simulink model "IEEE10_decommision"  (R2015b)
settings: Solver=FixedStepAuto  StartTime=0.0  StopTime=30  FixedStep=Ts  RelTol=1e-3
undefined symbols (not defined in the file): Cbase, Lbase, Ts, Xbase
libraries: powerlib x150, powerlib_meascontrol x27, simulink x9, sps_avr x3, powerlib_extras x1
(part 1 of 2)
settings Model: SimulationMode=accelerator  Creator=Eren  LastModifiedBy=Eren
settings DebuggingCC: UnconnectedInputMsg=none  UnconnectedOutputMsg=none  UnconnectedLineMsg=none

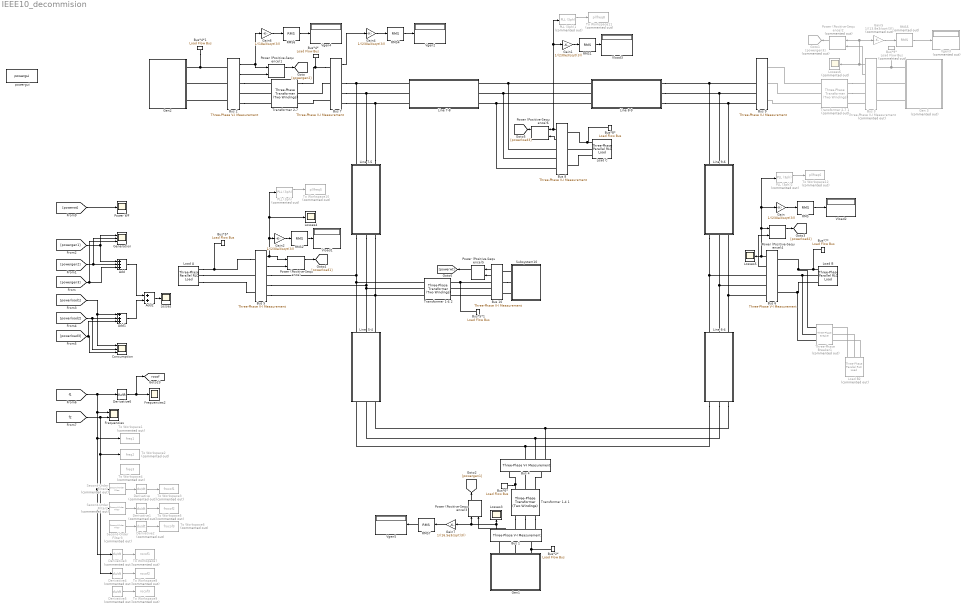
== system IEEE10_decommision ==
  Add : Sum  Inputs=3
  Add1 : Sum  Inputs=3
  Add2 : Sum
  Bus {1..2,4..10} (9 alike) : powerlib/Measurements/Three-Phase V-I Measurement  VoltageMeasurement=phase-to-ground  SetLabelV=off  LabelV=Vsabc  Vpu=off  VpuLL=on  CurrentMeasurement=yes  SetLabelI=off  LabelI=Isabc  Ipu=off  Pbase=100e6  Vbase=690  OutputType=Complex  PhasorSimulation=off  PSBequivalent=0
  Bus 3 : powerlib/Measurements/Three-Phase V-I Measurement  Commented=on  VoltageMeasurement=phase-to-ground  SetLabelV=off  LabelV=Vsabc  Vpu=off  VpuLL=on  CurrentMeasurement=yes  SetLabelI=off  LabelI=Isabc  Ipu=off  Pbase=100e6  Vbase=690  OutputType=Complex  PhasorSimulation=off  PSBequivalent=0
  Bus*2* : powerlib/Measurements/Load Flow Bus  LConnTagsString=a  Phases=single  Connectors=on one side  ID=Bus*1*  Vbase=16500  Vref=1.04  Vangle=0  VLF=1.04  VLFb=1  VLFc=1  angleLF=0  angleLFb=0  angleLFc=0
  Bus*4* : powerlib/Measurements/Load Flow Bus  LConnTagsString=a  Phases=single  Connectors=on one side  ID=Bus*7*  Vbase=230000  Vref=1  Vangle=0  VLF=1.027  VLFb=1  VLFc=1  angleLF=-1.988  angleLFb=0  angleLFc=0
  Bus*4*1 : powerlib/Measurements/Load Flow Bus  LConnTagsString=a  Phases=single  Connectors=on one side  ID=Bus*2*  Vbase=18e3  Vref=1.025  Vangle=0  VLF=1.025  VLFb=1  VLFc=1  angleLF=3.56  angleLFb=0  angleLFc=0
  Bus*5* : powerlib/Measurements/Load Flow Bus  LConnTagsString=a  Phases=single  Connectors=on one side  ID=Bus*5*  Vbase=230e3  Vref=1  Vangle=0  VLF=1.013  VLFb=1  VLFc=1  angleLF=-6.161  angleLFb=0  angleLFc=0
  Bus*5*1 : powerlib/Measurements/Load Flow Bus  LConnTagsString=a  Phases=single  Connectors=on one side  ID=Bus*10*  Vbase=690  Vref=1  Vangle=0  VLF=1.013  VLFb=1  VLFc=1  angleLF=-6.164  angleLFb=0  angleLFc=0
  Bus*6* : powerlib/Measurements/Load Flow Bus  LConnTagsString=a  Phases=single  Connectors=on one side  ID=Bus*4*  Vbase=230000  Vref=1  Vangle=0  VLF=1.034  VLFb=1  VLFc=1  angleLF=-4.035  angleLFb=0  angleLFc=0
  Bus*7* : powerlib/Measurements/Load Flow Bus  LConnTagsString=a  Phases=single  Connectors=on one side  ID=Bus*6*  Vbase=230e3  Vref=1  Vangle=0  VLF=1.022  VLFb=1  VLFc=1  angleLF=-8.159  angleLFb=0  angleLFc=0
  Bus*8* : powerlib/Measurements/Load Flow Bus  LConnTagsString=a  Phases=single  Connectors=on one side  ID=Bus*8*  Vbase=230e3  Vref=1  Vangle=0  VLF=1.018  VLFb=1  VLFc=1  angleLF=-6.531  angleLFb=0  angleLFc=0
  Bus*9* : powerlib/Measurements/Load Flow Bus  Commented=on  LConnTagsString=a  Phases=single  Connectors=on one side  ID=Bus*3*  Vbase=13800  Vref=1.025  Vangle=0  VLF=1.025  VLFb=1  VLFc=1  angleLF=6.455  angleLFb=0  angleLFc=0
  Concumption : Scope  NumInputPorts=3
  Derivative{,1..5} (6 alike) : Derivative  Commented=on
  Derivative6 : Derivative
  Frequencies : Scope  NumInputPorts=2
  Frequencies2 : Scope
  Gain{,1..2,4} (4 alike) : Gain  Gain=1/(230e3/sqrt(3))
  Gain5 : Gain  Commented=on  Gain=1/(13.8e3/sqrt(3))
  Gain6 : Gain  Gain=1/(18e3/sqrt(3))
  Gain7 : Gain  Gain=1/(16.5e3/sqrt(3))
  Gen 3 : Subsystem  Commented=on
  Gen1 : Subsystem
  Gen2 : Subsystem
  "Generation " : Scope  NumInputPorts=3
  Goto1 : Goto  Commented=on  GotoTag=powergen3
  Line  5-4 : Subsystem
  Line 6-4 : Subsystem
  Line 7-5 : Subsystem
  Line 7-8 : Subsystem
  Line 8-9 : Subsystem
  Line 9-6 : Subsystem
  Load A : powerlib/Elements/Three-Phase Parallel RLC Load  LConnTagsString=A|B|C  Configuration=Y (grounded)  NominalVoltage=(230000)*1.01282  Vabc=[1e3 1e3 1e3]  Vabcp=[1e3 1e3 1e3]  NominalFrequency=50  UnbalancedPower=off  ActivePower=125e6  InductivePower=50e6  CapacitivePower=0  Pabc=[10e3 9e3 11e3]  QLabc=[100 90 110]  QCabc=[100 90 110]  Pabcp=[10e3 9e3 11e3]  QLabcp=[100 90 110]  QCabcp=[100 90 110]  Measurements=None  LoadType=constant PQ
  Load B : powerlib/Elements/Three-Phase Parallel RLC Load  LConnTagsString=A|B|C  Configuration=Y (grounded)  NominalVoltage=(230000)*1.0221  Vabc=[1e3 1e3 1e3]  Vabcp=[1e3 1e3 1e3]  NominalFrequency=50  UnbalancedPower=off  ActivePower=90e6  InductivePower=30e6  CapacitivePower=0  Pabc=[10e3 9e3 11e3]  QLabc=[100 90 110]  QCabc=[100 90 110]  Pabcp=[10e3 9e3 11e3]  QLabcp=[100 90 110]  QCabcp=[100 90 110]  Measurements=None  LoadType=constant PQ
  Load B2 : powerlib/Elements/Three-Phase Parallel RLC Load  Commented=on  LConnTagsString=A|B|C  Configuration=Y (grounded)  NominalVoltage=230e3  Vabc=[1e3 1e3 1e3]  Vabcp=[1e3 1e3 1e3]  NominalFrequency=50  UnbalancedPower=off  ActivePower=31.5e6*2  InductivePower=0  CapacitivePower=0  Pabc=[10e3 9e3 11e3]  QLabc=[100 90 110]  QCabc=[100 90 110]  Pabcp=[10e3 9e3 11e3]  QLabcp=[100 90 110]  QCabcp=[100 90 110]  Measurements=None  LoadType=constant PQ
  Load C : powerlib/Elements/Three-Phase Parallel RLC Load  LConnTagsString=A|B|C  Configuration=Y (grounded)  NominalVoltage=(230000)*1.01809  Vabc=[1e3 1e3 1e3]  Vabcp=[1e3 1e3 1e3]  NominalFrequency=50  UnbalancedPower=off  ActivePower=100e6  InductivePower=35e6  CapacitivePower=0  Pabc=[10e3 9e3 11e3]  QLabc=[100 90 110]  QCabc=[100 90 110]  Pabcp=[10e3 9e3 11e3]  QLabcp=[100 90 110]  QCabcp=[100 90 110]  Measurements=None  LoadType=constant PQ
  "Losses " : Scope
  Losses3 : Scope
  Losses4 : Scope
  Losses5 : Scope
  Losses6 : Scope  Commented=on
  PLL (3ph) : powerlib_meascontrol/PLL/PLL (3ph)  Commented=on  Fmin=45  Par_Init=[0, 50]  ParK=[180, 3200, 1]  TcD=1e-4  MaxRateChangeFreq=12  FilterCutOffFreq=25  Ts=0  AGC=on
  PLL (3ph)1 : powerlib_meascontrol/PLL/PLL (3ph)  Commented=on  Fmin=45  Par_Init=[0, 50]  ParK=[180, 3200, 1]  TcD=1e-4  MaxRateChangeFreq=12  FilterCutOffFreq=25  Ts=0  AGC=on
  PLL (3ph)2 : powerlib_meascontrol/PLL/PLL (3ph)  Commented=on  Fmin=45  Par_Init=[0, 50]  ParK=[180, 3200, 1]  TcD=1e-4  MaxRateChangeFreq=12  FilterCutOffFreq=25  Ts=0  AGC=on
  Power (Positive-Sequence){,1,3..6} (6 alike) : powerlib_meascontrol/Measurements/Power (Positive-Sequence)  Freq=50  Vinit=[0, 0]  Iinit=[0, 0]  Ts=0
  Power (Positive-Sequence)2 : powerlib_meascontrol/Measurements/Power (Positive-Sequence)  Commented=on  Freq=50  Vinit=[0, 0]  Iinit=[0, 0]  Ts=0
  Power WF : Scope
  RMS{,1..2,4,6..7} (6 alike) : powerlib_meascontrol/Measurements/RMS  TrueRMS=on  Freq=50  RMSInit=120  Ts=0
  RMS5 : powerlib_meascontrol/Measurements/RMS  Commented=on  TrueRMS=on  Freq=50  RMSInit=120  Ts=0
  Second-Order Filter1 : powerlib_meascontrol/Filters/Second-Order Filter  Commented=on  FilterType=Lowpass  Fo=2  Zeta=0.707  Ts=0  Initialize=off  Vac_Init="[0,  0,  60]"  Vdc_Init=0  PlotResponse=off  FreqRange=[0, 500, 1]
  Second-Order Filter2 : powerlib_meascontrol/Filters/Second-Order Filter  Commented=on  FilterType=Lowpass  Fo=2  Zeta=0.707  Ts=0  Initialize=off  Vac_Init="[0,  0,  60]"  Vdc_Init=0  PlotResponse=off  FreqRange=[0, 500, 1]
  Second-Order Filter3 : powerlib_meascontrol/Filters/Second-Order Filter  Commented=on  FilterType=Lowpass  Fo=2  Zeta=0.707  Ts=0  Initialize=off  Vac_Init="[0,  0,  60]"  Vdc_Init=0  PlotResponse=off  FreqRange=[0, 500, 1]
  Subsystem10 : Subsystem
  Three-Phase Breaker1 : powerlib/Elements/Three-Phase Breaker  Commented=on  InitialState=open  SwitchA=on  SwitchB=on  SwitchC=on  SwitchTimes=loadconnection  External=off  BreakerResistance=0.01  SnubberResistance=1e6  SnubberCapacitance=inf  Measurements=None
  To Workspace1 : ToWorkspace  Commented=on  VariableName=freq1  SaveFormat=Timeseries  SampleTime=-1
  To Workspace10 : ToWorkspace  Commented=on  VariableName=pllfreq5  SaveFormat=Timeseries  SampleTime=-1
  To Workspace11 : ToWorkspace  Commented=on  VariableName=pllfreq8  SaveFormat=Timeseries  SampleTime=-1
  To Workspace12 : ToWorkspace  Commented=on  VariableName=pllfreq6  SaveFormat=Timeseries  SampleTime=-1
  To Workspace2 : ToWorkspace  Commented=on  VariableName=freq2  SaveFormat=Timeseries  SampleTime=-1
  To Workspace3 : ToWorkspace  Commented=on  VariableName=frocof1  SaveFormat=Timeseries  SampleTime=-1
  To Workspace4 : ToWorkspace  Commented=on  VariableName=freq3  SaveFormat=Timeseries  SampleTime=-1
  To Workspace5 : ToWorkspace  Commented=on  VariableName=frocof2  SaveFormat=Timeseries  SampleTime=-1
  To Workspace6 : ToWorkspace  Commented=on  VariableName=frocof3  SaveFormat=Timeseries  SampleTime=-1
  To Workspace7 : ToWorkspace  Commented=on  VariableName=rocof1  SaveFormat=Timeseries  SampleTime=-1
  To Workspace8 : ToWorkspace  Commented=on  VariableName=rocof2  SaveFormat=Timeseries  SampleTime=-1
  To Workspace9 : ToWorkspace  Commented=on  VariableName=rocof3  SaveFormat=Timeseries  SampleTime=-1
  Transformer 1-4 1 : powerlib/Elements/Three-Phase Transformer (Two Windings)  Winding1Connection=Yg  Winding2Connection=Yg  CoreType=Three single-phase transformers  SetSaturation=off  Hysteresis=off  DataFile='hysteresis'  SetInitialFlux=off  Measurements=None  UNITS=pu  NominalPower=[ 250e6 , 50 ]  Winding1=[ 16.5e3 , 0.00001 , 0.144/2 ]  Winding2="[ 230e3 , 0.00001  , 0.144/2 ]"  Rm=500  Lm=500  L0=0.5  Saturation=[ 0,0 ; 0.0024,1.2 ; 1.0,1.52 ]  InitialFluxes=[ 0.8 , -0.8 , 0.7 ]  MoreParameters=off  BreakLoop=off  DataType=off  TransfoNumber=1
  Transformer 1-4 2 : powerlib/Elements/Three-Phase Transformer (Two Windings)  Winding1Connection=Yg  Winding2Connection=Yg  CoreType=Three single-phase transformers  SetSaturation=off  Hysteresis=off  DataFile='hysteresis'  SetInitialFlux=off  Measurements=None  UNITS=pu  NominalPower=[ 50e6 , 50 ]  Winding1=[ 690 , 0.00001 , 0.05/2 ]  Winding2="[ 230e3 , 0.00001  , 0.05/2 ]"  Rm=500  Lm=500  L0=0.5  Saturation=[ 0,0 ; 0.0024,1.2 ; 1.0,1.52 ]  InitialFluxes=[ 0.8 , -0.8 , 0.7 ]  MoreParameters=off  BreakLoop=off  DataType=off  TransfoNumber=1
  "Transformer 2-7 " : powerlib/Elements/Three-Phase Transformer (Two Windings)  Winding1Connection=Yg  Winding2Connection=Yg  CoreType=Three single-phase transformers  SetSaturation=off  Hysteresis=off  DataFile='hysteresis'  SetInitialFlux=off  Measurements=None  UNITS=pu  NominalPower=[ 200e6 , 50 ]  Winding1=[18000 1e-05 0.0625]  Winding2=[2.3e+05 1e-05 0.0625]  Rm=500  Lm=500  L0=0.5  Saturation=[0 0;0.0024 1.2;1 1.52]  InitialFluxes=[0.79999 -0.79999 0.69999]  MoreParameters=off  BreakLoop=off  DataType=off  TransfoNumber=1
  Transformer 2-7 1 : powerlib/Elements/Three-Phase Transformer (Two Windings)  Commented=on  Winding1Connection=Yg  Winding2Connection=Yg  CoreType=Three single-phase transformers  SetSaturation=off  Hysteresis=off  DataFile='hysteresis'  SetInitialFlux=off  Measurements=None  UNITS=pu  NominalPower=[ 150e6 , 50 ]  Winding1="[ 13.8e3 , 0.00001 , 0.0879/2  ]"  Winding2="[ 230e3 , 0.00001  , 0.0879/2 ]"  Rm=500  Lm=500  L0=0.5  Saturation=[ 0,0 ; 0.0024,1.2 ; 1.0,1.52 ]  InitialFluxes=[ 0.8 , -0.8 , 0.7 ]  MoreParameters=off  BreakLoop=off  DataType=off  TransfoNumber=1
  Vgen2 : Display
      settings: Decimation=5
  Vgen3 : Display  Commented=on
      settings: Decimation=5
  Vgen4 : Display
      settings: Decimation=5
  Vgen5 : Display
      settings: Decimation=5
  Vload1 : Display
      settings: Decimation=5
  Vload2 : Display
      settings: Decimation=5
  Vload3 : Display
      settings: Decimation=5
  powergui : powerlib/powergui  Priority=2  SimulationMode=Discrete  SolverType=Tustin  SampleTime=Ts  frequency=50  SPID=on  DisableSnubberDevices=on  DisableRonSwitches=on  DisableVfSwitches=on  SwTol=0  DisplayEquations=off  Interpol=off  ExternalGateDelay=off  methode=off  Ts=0  FunctionMessages=off  echomessages=off  HookPort=off  EnableUseOfTLC=off  x0status=steady  frequencyindice=50  Pbase=100e6  ErrMax=0.0001  Iterations=50  UnitsV=kV  UnitsW=MW  buscounter=10  RestoreLinks=warning  ResistiveCurrentMeasurement=off  Frange=[0:2:500]  Ylog=off  Xlog=on  ShowGrid=off  save=off  variable=ZData  structure=0  ZoomFFT=on  StartTime=0.0  cycles=1  DisplayStyle=1  fundamental=60  FreqAxis=off  MaxFrequency=1000  frequencyindicesteady=1  RmsSteady=2  display=off
  tag scope: rocof=global
  wires:
  Bus 5/2 -> Power (Positive-Sequence)/2
  Power (Positive-Sequence)/1 -> [powerload1]
  Bus 2/2 -> Power (Positive-Sequence)1/2
  Bus 3/2 -> Power (Positive-Sequence)2/2
  Bus 1/2 -> Power (Positive-Sequence)3/2
  Power (Positive-Sequence)1/1 -> [powergen2]
  Power (Positive-Sequence)2/1 -> Goto1/1
  Power (Positive-Sequence)3/1 -> [powergen1]
  Bus 6/2 -> Power (Positive-Sequence)4/2
  Power (Positive-Sequence)4/1 -> [powerload2]
  [powergen1] -> "Generation "/1, Add/1
  [powergen2] -> Add/2, "Generation "/2
  [powergen3] -> "Generation "/3, Add/3
  [powerload1] -> Add1/1, Concumption/1
  [powerload2] -> Add1/2, Concumption/2
  [powerload3] -> Add1/3, Concumption/3
  Add/1 -> Add2/1
  Add1/1 -> Add2/2
  Add2/1 -> "Losses "/1
  Bus 8/2 -> Power (Positive-Sequence)6/2
  Power (Positive-Sequence)6/1 -> [powerload3]
  RMS/1 -> Vload2/1
  Gain/1 -> RMS/1
  RMS1/1 -> Vload3/1
  Gain1/1 -> RMS1/1
  Bus 5/1 -> Power (Positive-Sequence)/1, PLL (3ph)/1, Losses4/1, Gain2/1
  RMS2/1 -> Vload1/1
  Gain2/1 -> RMS2/1
  Bus 1/1 -> Gain7/1, Power (Positive-Sequence)3/1, Losses3/1
  RMS4/1 -> Vgen2/1
  Gain4/1 -> RMS4/1
  Bus 3/1 -> Power (Positive-Sequence)2/1, Gain5/1, Losses6/1
  Bus 7/1 -> Gain4/1
  RMS6/1 -> Vgen4/1
  Gain6/1 -> RMS6/1
  Bus 2/1 -> Gain6/1, Power (Positive-Sequence)1/1
  RMS7/1 -> Vgen5/1
  Gain7/1 -> RMS7/1
  [f2] -> Derivative4/1, Second-Order Filter2/1, To Workspace2/1, Frequencies/2
  Second-Order Filter1/1 -> Derivative/1
  Second-Order Filter2/1 -> Derivative1/1
  Second-Order Filter3/1 -> Derivative2/1
  Gain5/1 -> RMS5/1
  RMS5/1 -> Vgen3/1
  [f1] -> Derivative3/1, Second-Order Filter1/1, To Workspace1/1, Frequencies/1, Derivative6/1
  Derivative/1 -> To Workspace3/1
  Derivative1/1 -> To Workspace5/1
  Derivative2/1 -> To Workspace6/1
  Derivative3/1 -> To Workspace7/1
  Derivative4/1 -> To Workspace8/1
  Derivative5/1 -> To Workspace9/1
  PLL (3ph)/1 -> To Workspace10/1
  Bus 8/1 -> PLL (3ph)1/1, Gain1/1, Power (Positive-Sequence)6/1
  PLL (3ph)1/1 -> To Workspace11/1
  Bus 6/1 -> Gain/1, PLL (3ph)2/1, Power (Positive-Sequence)4/1, Losses5/1
  PLL (3ph)2/1 -> To Workspace12/1
  Derivative6/1 -> [rocof], Frequencies2/1
  Bus 10/1 -> Power (Positive-Sequence)5/1
  Bus 10/2 -> Power (Positive-Sequence)5/2
  Power (Positive-Sequence)5/1 -> [powerwt]
  [powerwt] -> Power WF/1
  connections:
  Bus 5/RConn1 -- Transformer 1-4 2/RConn1 -- Line  5-4/LConn1 -- Line 7-5/RConn1
  Bus 5/RConn2 -- Line 7-5/RConn2 -- Transformer 1-4 2/RConn2 -- Line  5-4/LConn2
  Bus 5/RConn3 -- Line 7-5/RConn3 -- Transformer 1-4 2/RConn3 -- Line  5-4/LConn3
  Line 6-4/RConn1 -- Bus 4/RConn1 -- Line  5-4/RConn1
  Line  5-4/RConn2 -- Bus 4/RConn2 -- Line 6-4/RConn2
  Line 6-4/RConn3 -- Bus 4/RConn3 -- Line  5-4/RConn3
  Bus 6/RConn1 -- Line 9-6/RConn1 -- Line 6-4/LConn1
  Line 9-6/RConn3 -- Line 6-4/LConn3 -- Bus 6/RConn3
  Line 9-6/RConn2 -- Line 6-4/LConn2 -- Bus 6/RConn2
  Bus 9/RConn1 -- Line 8-9/RConn1 -- Line 9-6/LConn1
  Bus 9/RConn2 -- Line 8-9/RConn2 -- Line 9-6/LConn2
  Bus 9/RConn3 -- Line 8-9/RConn3 -- Line 9-6/LConn3
  Line 8-9/LConn1 -- Line 7-8/RConn1 -- Bus 8/RConn1
  Line 8-9/LConn2 -- Bus 8/RConn2 -- Line 7-8/RConn2
  Line 8-9/LConn3 -- Bus 8/RConn3 -- Line 7-8/RConn3
  Bus 7/RConn1 -- Line 7-8/LConn1 -- Line 7-5/LConn1
  Line 7-5/LConn2 -- Line 7-8/LConn2 -- Bus 7/RConn2
  Line 7-5/LConn3 -- Line 7-8/LConn3 -- Bus 7/RConn3
  Gen 3/RConn1 -- Bus*9*/LConn1 -- Bus 3/LConn1
  Bus*4*1/LConn1 -- Gen2/RConn1 -- Bus 2/LConn1
  Bus 7/LConn1 -- "Transformer 2-7 "/RConn1 -- Bus*4*/LConn1
  Transformer 1-4 1/LConn2 -- Bus 1/RConn2
  Bus*6*/LConn1 -- Bus 4/LConn1 -- Transformer 1-4 1/RConn1
  Transformer 1-4 1/RConn2 -- Bus 4/LConn2
  Bus 7/LConn3 -- "Transformer 2-7 "/RConn3
  Gen1/RConn3 -- Bus*2*/LConn1 -- Bus 1/LConn3
  Gen 3/RConn3 -- Bus 3/LConn3
  Transformer 1-4 1/LConn3 -- Bus 1/RConn3
  Transformer 2-7 1/RConn2 -- Bus 9/LConn2
  Bus 5/LConn1 -- Load A/LConn1 -- Bus*5*/LConn1
  Load B/LConn2 -- Three-Phase Breaker1/LConn2 -- Bus 6/LConn2
  Load A/LConn2 -- Bus 5/LConn2
  Transformer 2-7 1/RConn3 -- Bus 9/LConn3
  Transformer 2-7 1/RConn1 -- Bus 9/LConn1
  Load B/LConn3 -- Three-Phase Breaker1/LConn3 -- Bus 6/LConn3
  Load B/LConn1 -- Bus*7*/LConn1 -- Bus 6/LConn1 -- Three-Phase Breaker1/LConn1
  Gen1/RConn2 -- Bus 1/LConn2
  Load A/LConn3 -- Bus 5/LConn3
  Transformer 2-7 1/LConn2 -- Bus 3/RConn2
  Transformer 2-7 1/LConn1 -- Bus 3/RConn1
  Bus 7/LConn2 -- "Transformer 2-7 "/RConn2
  Gen1/RConn1 -- Bus 1/LConn1
  Transformer 1-4 1/RConn3 -- Bus 4/LConn3
  Gen 3/RConn2 -- Bus 3/LConn2
  Transformer 1-4 1/LConn1 -- Bus 1/RConn1
  Bus 3/RConn3 -- Transformer 2-7 1/LConn3
  Bus 8/LConn1 -- Bus*8*/LConn1 -- Load C/LConn1
  Load C/LConn2 -- Bus 8/LConn2
  Load C/LConn3 -- Bus 8/LConn3
  Load B2/LConn1 -- Three-Phase Breaker1/RConn1
  Load B2/LConn3 -- Three-Phase Breaker1/RConn3
  Load B2/LConn2 -- Three-Phase Breaker1/RConn2
  Bus 2/LConn2 -- Gen2/RConn2
  Bus 2/LConn3 -- Gen2/RConn3
  Bus 2/RConn3 -- "Transformer 2-7 "/LConn3
  "Transformer 2-7 "/LConn2 -- Bus 2/RConn2
  Bus 2/RConn1 -- "Transformer 2-7 "/LConn1
  Bus 10/RConn1 -- Bus*5*1/LConn1 -- Transformer 1-4 2/LConn1
  Bus 10/RConn2 -- Transformer 1-4 2/LConn2
  Bus 10/RConn3 -- Transformer 1-4 2/LConn3
  Subsystem10/RConn3 -- Bus 10/LConn3
  Subsystem10/RConn1 -- Bus 10/LConn1
  Bus 10/LConn2 -- Subsystem10/RConn2

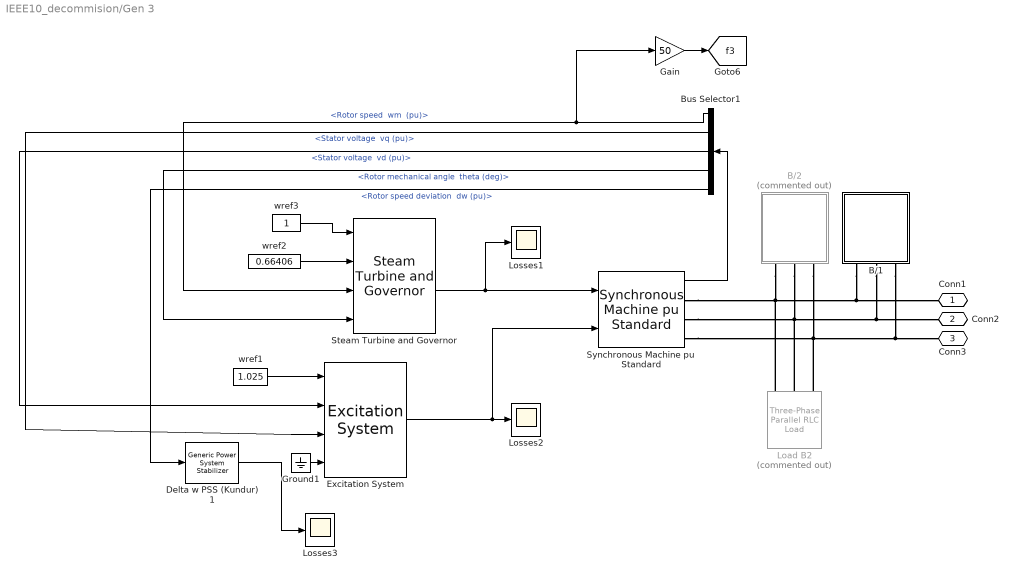
== system IEEE10_decommision/Gen 3 ==
  B/1 : Subsystem
  B/2 : Subsystem  Commented=on
  Bus Selector1 : BusSelector  OutputSignals="Mechanical.Rotor speed  wm  (pu),dq0 components.Stator voltage  vq (pu),dq0 components.Stator voltage  vd (pu),Mechanical.Rotor mechanical angle  theta (deg),Mechanical.Rotor speed deviation  dw (pu)"
  Delta w PSS (Kundur) 1 : powerlib/Machines/Generic Power System Stabilizer  Tsensor=30e-3  K=10  Twashout=10  Tleadlag1=[50e-3 20e-3]  Tleadlag2=[3 5.4]  VSlimits=[-0.15 0.15]  Vinit=0  Plot_On=off  MagdB_On=off  FreqRange=logspace(-2,2,500)
  Excitation System : sps_avr/Excitation System  tr=20e-3  reg=[ 350, 0.001 ]  exc=[ 1, 0 ]  tgr=[ 0, 0 ]  damp=[ 0.001, 0.1 ]  sat=[ 0, 0 ]  lim=[ -11.5, 11.5, 0 ]  v0=[1.025 1.4054]
  Gain : Gain  Gain=50
  Ground1 : Ground
  Load B2 : powerlib/Elements/Three-Phase Parallel RLC Load  Commented=on  LConnTagsString=A|B|C  Configuration=Y (grounded)  NominalVoltage=(13800)*1.025  Vabc=[1e3 1e3 1e3]  Vabcp=[1e3 1e3 1e3]  NominalFrequency=50  UnbalancedPower=off  ActivePower=0.64e6  InductivePower=0  CapacitivePower=0  Pabc=[10e3 9e3 11e3]  QLabc=[100 90 110]  QCabc=[100 90 110]  Pabcp=[10e3 9e3 11e3]  QLabcp=[100 90 110]  QCabcp=[100 90 110]  Measurements=None  LoadType=constant PQ
  Losses1 : Scope
  Losses2 : Scope
  Losses3 : Scope
  Steam Turbine and Governor : powerlib/Machines/Steam Turbine and Governor  gentype=Tandem-compound (single mass)  reg1="[ 1  0.05    0 ]"  reg2="[ 0.001  0.3 ]"  reg3="[ -0.1  0.1  0  4.496]"  N=3000  turb1="[ 0  10   3.3   0.5   ]"  turb2="[ 0.5   0.5   0  0 ]"  HA="[  1.5498   0.24894  0  0 ]"  KA="[  83.47  42.702  0  0 ]"  DA="[  0.3104  0.05  0  0 ]*8"  ini1=0.66406  ini2=[0.5,-120.13]
  Synchronous Machine pu Standard : powerlib/Machines/Synchronous Machine pu Standard  PresetModel=No  MechanicalLoad=Mechanical power Pm  ShowDetailedParameters=on  RotorType=Round  Units=per unit standard parameters  MeasurementBus=off  NominalParameters=[128e+06 13.8e3 50]  Reactances1=[ 1.68, 0.232064, 0.2, 1.609984, 0.32, 0.2, 0.094976 ]  Reactances2=[2.24 0.17 0.12 1.02 0.13 0.08]  dAxisTimeConstants=Short-circuit  qAxisTimeConstants=Short-circuit  TimeConstants1="[ 4.4849  0.0681  0.1  ]"  TimeConstants2=[ 8.0, 0.03, 1.0, 0.07 ]  TimeConstants3="[  4.49  0.0681  0.0513  ]"  TimeConstants4=[ 8.0, 0.03, 0.3371, 0.0295 ]  TimeConstants5=[ 1.01, 0.053, 0.1 ]  TimeConstants6=[ 1.3201, 0.023, 1.0, 0.07 ]  TimeConstants7=[0.012 0.003 0.003]  TimeConstants8=[ 5.89, 0.0575, 0.6, 0.08 ]  StatorResistance=0.0000000107875  Mechanical=[2.35 0.02056 2]  PolePairs=20  InitialConditions=[0 -34.1885 0.65285 0.65285 0.65285 13.5391 -106.461 133.539 1.40539]  SetSaturation=off  Saturation=[0.6404,0.7127,0.8441,0.9214,0.9956,1.082,1.19,1.316,1.457;0.7,0.7698,0.8872,0.9466,0.9969,1.046,1.1,1.151,1.201]  LoadFlowParameters=[1 85000000 0 0 0]  TsPowergui=0  TsBlock=-1  IterativeModel=Trapezoidal non iterative  BusType=PV  Pref=85e6  Qref=0  Qmin=-inf  Qmax=inf  PLF=0  QLF=0
  wref1 : Constant  Value=1.025
  wref2 : Constant  Value=0.66406
  wref3 : Constant
  Conn1 : PMIOPort  Port=1  Side=Right
  Conn2 : PMIOPort  Port=2  Side=Right
  Conn3 : PMIOPort  Port=3  Side=Right
  tag scope: f3=global
  wires:
  Gain/1 -> [f3]
  Bus Selector1/2 -> Excitation System/3  "<Stator voltage  vq (pu)>"
  Bus Selector1/1 -> Gain/1, Steam Turbine and Governor/3  "<Rotor speed  wm  (pu)>"
  Bus Selector1/3 -> Excitation System/2  "<Stator voltage  vd (pu)>"
  Excitation System/1 -> Losses2/1, Synchronous Machine pu Standard/2
  Delta w PSS (Kundur) 1/1 -> Losses3/1
  wref1/1 -> Excitation System/1
  Synchronous Machine pu Standard/1 -> Bus Selector1/1
  wref3/1 -> Steam Turbine and Governor/1
  wref2/1 -> Steam Turbine and Governor/2
  Bus Selector1/4 -> Steam Turbine and Governor/4  "<Rotor mechanical angle  theta (deg)>"
  Steam Turbine and Governor/3 -> Losses1/1, Synchronous Machine pu Standard/1
  Bus Selector1/5 -> Delta w PSS (Kundur) 1/1  "<Rotor speed deviation  dw (pu)>"
  Ground1/1 -> Excitation System/4
  connections:
  Synchronous Machine pu Standard/RConn1 -- B/1/RConn1 -- Conn1/RConn1 -- B/2/RConn1 -- Load B2/LConn1
  Synchronous Machine pu Standard/RConn2 -- B/1/RConn2 -- Conn2/RConn1 -- B/2/RConn2 -- Load B2/LConn2
  Synchronous Machine pu Standard/RConn3 -- B/1/RConn3 -- Conn3/RConn1 -- B/2/RConn3 -- Load B2/LConn3

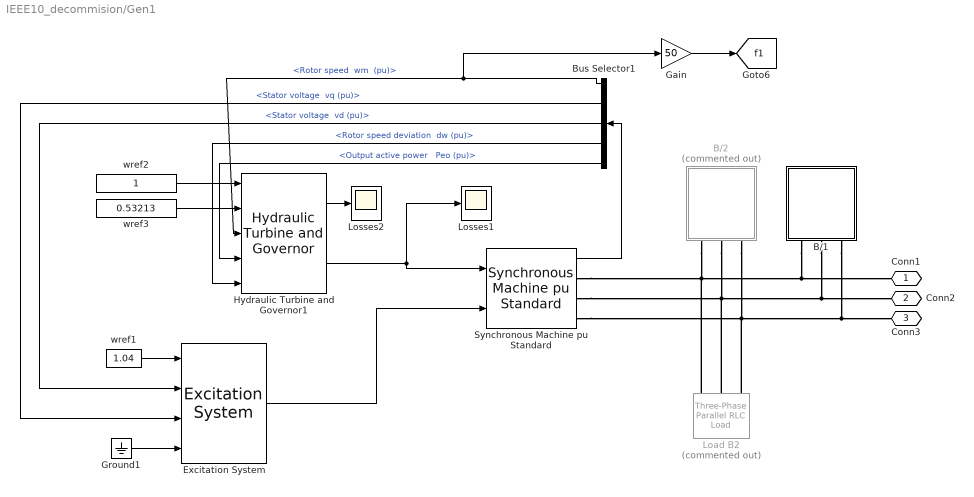
== system IEEE10_decommision/Gen1 ==
  B/1 : Subsystem
  B/2 : Subsystem  Commented=on
  Bus Selector1 : BusSelector  OutputSignals="Mechanical.Rotor speed  wm  (pu),dq0 components.Stator voltage  vq (pu),dq0 components.Stator voltage  vd (pu),Mechanical.Rotor speed deviation  dw (pu),Output active power   Peo (pu)"
  Excitation System : sps_avr/Excitation System  tr=20e-3  reg=[ 350, 0.001 ]  exc=[ 1, 0 ]  tgr=[ 0, 0 ]  damp=[ 0.001, 0.1 ]  sat=[ 0, 0 ]  lim=[ -11.5, 11.5, 0 ]  v0=[1.04 1.4418]
  Gain : Gain  Gain=50
  Ground1 : Ground
  Hydraulic Turbine and Governor1 : powerlib/Machines/Hydraulic Turbine and Governor  sm="[ 10/3  0.07 ]"  gate="[  0.01  0.97518  -0.1  0.1 ]"  reg="[  0.05  1.163  0.105  0  0.01  ]"  hyd="[  0  2.67*2  ]"  dref=0  po=0.53345
  Load B2 : powerlib/Elements/Three-Phase Parallel RLC Load  Commented=on  LConnTagsString=A|B|C  Configuration=Y (grounded)  NominalVoltage=(16500)*1.04  Vabc=[1e3 1e3 1e3]  Vabcp=[1e3 1e3 1e3]  NominalFrequency=50  UnbalancedPower=off  ActivePower=1.2375e6  InductivePower=0  CapacitivePower=0  Pabc=[10e3 9e3 11e3]  QLabc=[100 90 110]  QCabc=[100 90 110]  Pabcp=[10e3 9e3 11e3]  QLabcp=[100 90 110]  QCabcp=[100 90 110]  Measurements=None  LoadType=constant PQ
  Losses1 : Scope
  Losses2 : Scope
  Synchronous Machine pu Standard : powerlib/Machines/Synchronous Machine pu Standard  PresetModel=No  MechanicalLoad=Mechanical power Pm  ShowDetailedParameters=on  RotorType=Round  Units=per unit standard parameters  MeasurementBus=off  NominalParameters=[247.5e+06 16.5e3 50]  Reactances1=[1.719936 0.230016 0.2 1.65984 0.378048 0.2 0.100032]  Reactances2=[0.3614 0.1505 0.1 0.2398275 0.1 0.0832]  dAxisTimeConstants=Short-circuit  qAxisTimeConstants=Short-circuit  TimeConstants1="[ 4.4849  0.0681  0.1  ]"  TimeConstants2=[ 8.0, 0.03, 1.0, 0.07 ]  TimeConstants3="[  4.49  0.0681  0.0513  ]"  TimeConstants4=[ 8.0, 0.03, 0.3371, 0.0295 ]  TimeConstants5=[ 1.01, 0.053, 0.1 ]  TimeConstants6=[ 1.3201, 0.023, 1.0, 0.07 ]  TimeConstants7=[8.96 0.0575 0.0945]  TimeConstants8=[ 6 0.0575 0.535 0.0945]  StatorResistance=0.005  Mechanical=[9.5515 0.02056 20]  PolePairs=20  InitialConditions=[0 -53.3005 0.514948 0.514948 0.514948 -6.47972 -126.48 113.52 1.44178]  SetSaturation=off  Saturation=[0.6404,0.7127,0.8441,0.9214,0.9956,1.082,1.19,1.316,1.457;0.7,0.7698,0.8872,0.9466,0.9969,1.046,1.1,1.151,1.201]  LoadFlowParameters=[2 100000000 17160 0 0]  TsPowergui=0  TsBlock=-1  IterativeModel=Trapezoidal non iterative  BusType=swing  Pref=50e6  Qref=0  Qmin=-inf  Qmax=inf  PLF=0  QLF=0
  wref1 : Constant  Value=1.04
  wref2 : Constant
  wref3 : Constant  Value=0.53213
  Conn1 : PMIOPort  Port=1  Side=Right
  Conn2 : PMIOPort  Port=2  Side=Right
  Conn3 : PMIOPort  Port=3  Side=Right
  tag scope: f1=global
  wires:
  Gain/1 -> [f1]
  Bus Selector1/2 -> Excitation System/3  "<Stator voltage  vq (pu)>"
  Bus Selector1/1 -> Hydraulic Turbine and Governor1/3, Gain/1  "<Rotor speed  wm  (pu)>"
  Bus Selector1/3 -> Excitation System/2  "<Stator voltage  vd (pu)>"
  Excitation System/1 -> Synchronous Machine pu Standard/2
  wref1/1 -> Excitation System/1
  Synchronous Machine pu Standard/1 -> Bus Selector1/1
  Bus Selector1/4 -> Hydraulic Turbine and Governor1/5  "<Rotor speed deviation  dw (pu)>"
  Hydraulic Turbine and Governor1/2 -> Synchronous Machine pu Standard/1, Losses1/1
  wref2/1 -> Hydraulic Turbine and Governor1/1
  Hydraulic Turbine and Governor1/1 -> Losses2/1
  wref3/1 -> Hydraulic Turbine and Governor1/2
  Bus Selector1/5 -> Hydraulic Turbine and Governor1/4  "<Output active power   Peo (pu)>"
  Ground1/1 -> Excitation System/4
  connections:
  Synchronous Machine pu Standard/RConn1 -- Load B2/LConn1 -- B/1/RConn1 -- Conn1/RConn1 -- B/2/RConn1
  Synchronous Machine pu Standard/RConn2 -- Load B2/LConn2 -- B/1/RConn2 -- Conn2/RConn1 -- B/2/RConn2
  Synchronous Machine pu Standard/RConn3 -- Load B2/LConn3 -- B/1/RConn3 -- Conn3/RConn1 -- B/2/RConn3

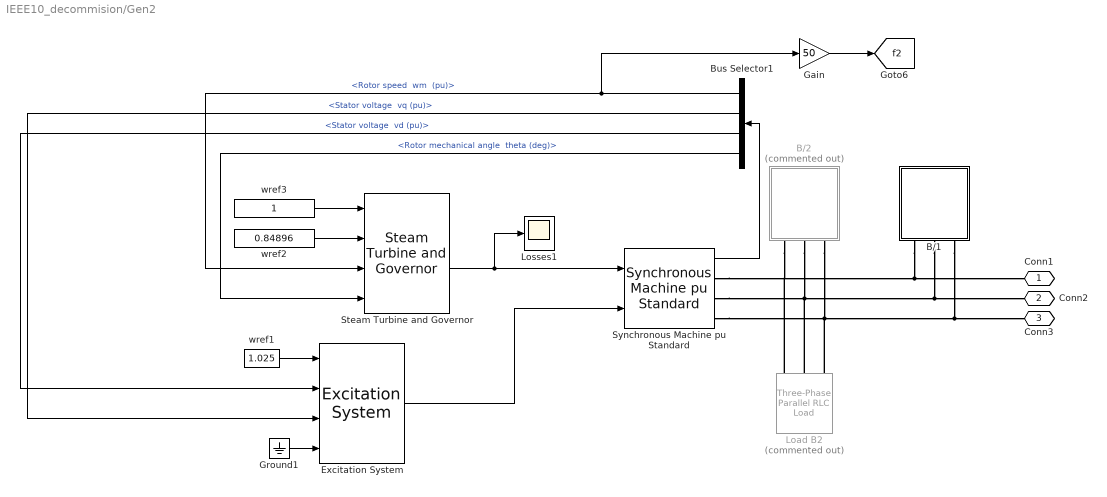
== system IEEE10_decommision/Gen2 ==
  B/1 : Subsystem
  B/2 : Subsystem  Commented=on
  Bus Selector1 : BusSelector  OutputSignals="Mechanical.Rotor speed  wm  (pu),dq0 components.Stator voltage  vq (pu),dq0 components.Stator voltage  vd (pu),Mechanical.Rotor mechanical angle  theta (deg)"
  Excitation System : sps_avr/Excitation System  tr=20e-3  reg=[ 350, 0.001 ]  exc=[ 1, 0 ]  tgr=[ 0, 0 ]  damp=[ 0.001, 0.1 ]  sat=[ 0, 0 ]  lim=[ -11.5, 11.5, 0 ]  v0=[1.025 1.784]
  Gain : Gain  Gain=50
  Ground1 : Ground
  Load B2 : powerlib/Elements/Three-Phase Parallel RLC Load  Commented=on  LConnTagsString=A|B|C  Configuration=Y (grounded)  NominalVoltage=(18000)*1.025  Vabc=[1e3 1e3 1e3]  Vabcp=[1e3 1e3 1e3]  NominalFrequency=50  UnbalancedPower=off  ActivePower=0.96e6  InductivePower=0  CapacitivePower=0  Pabc=[10e3 9e3 11e3]  QLabc=[100 90 110]  QCabc=[100 90 110]  Pabcp=[10e3 9e3 11e3]  QLabcp=[100 90 110]  QCabcp=[100 90 110]  Measurements=None  LoadType=constant PQ
  Losses1 : Scope
  Steam Turbine and Governor : powerlib/Machines/Steam Turbine and Governor  gentype=Tandem-compound (single mass)  reg1="[ 1  0.05    0 ]"  reg2="[ 0.001  0.3 ]"  reg3="[ -0.1  0.1  0  4.496]"  N=3000  turb1="[ 0  10   3.3   0.5   ]"  turb2="[ 0.5   0.5   0  0 ]"  HA="[  1.5498   0.24894  0  0 ]"  KA="[  83.47  42.702  0  0 ]"  DA="[  0.3104  0.05  0  0 ]*8"  ini1=0.85239  ini2=170/192,-120.13]
  Synchronous Machine pu Standard : powerlib/Machines/Synchronous Machine pu Standard  PresetModel=No  MechanicalLoad=Mechanical power Pm  ShowDetailedParameters=on  RotorType=Round  Units=per unit standard parameters  MeasurementBus=off  NominalParameters=[192e+06 18e3 50]  Reactances1=[1.719936 0.230016 0.2 1.65984 0.378048 0.2 0.100032]  Reactances2=[1.719936 0.230016 0.2 1.65984 0.100032]  dAxisTimeConstants=Short-circuit  qAxisTimeConstants=Short-circuit  TimeConstants1="[ 4.4849  0.0681  0.1  ]"  TimeConstants2=[ 8.0, 0.03, 1.0, 0.07 ]  TimeConstants3="[  4.49  0.0681  0.0513  ]"  TimeConstants4=[ 8.0, 0.03, 0.3371, 0.0295 ]  TimeConstants5=[ 1.01, 0.053, 0.1 ]  TimeConstants6=[ 1.3201, 0.023, 1.0, 0.07 ]  TimeConstants7=[6 0.0575 0.0945]  TimeConstants8=[ 6 0.0575 0.535 0.0945]  StatorResistance=0.005  Mechanical=[3.9216 0.02056 2]  PolePairs=20  InitialConditions=[0 -34.4122 0.828672 0.828672 0.828672 1.73652 -118.263 121.737 1.78399]  SetSaturation=off  Saturation=[0.6404,0.7127,0.8441,0.9214,0.9956,1.082,1.19,1.316,1.457;0.7,0.7698,0.8872,0.9466,0.9969,1.046,1.1,1.151,1.201]  LoadFlowParameters=[1 163000000 18450 0 0]  TsPowergui=0  TsBlock=-1  IterativeModel=Trapezoidal non iterative  BusType=PV  Pref=163e6  Qref=0  Qmin=-inf  Qmax=inf  PLF=0  QLF=0
  wref1 : Constant  Value=1.025
  wref2 : Constant  Value=0.84896
  wref3 : Constant
  Conn1 : PMIOPort  Port=1  Side=Right
  Conn2 : PMIOPort  Port=2  Side=Right
  Conn3 : PMIOPort  Port=3  Side=Right
  tag scope: f2=global
  wires:
  Gain/1 -> [f2]
  Bus Selector1/2 -> Excitation System/3  "<Stator voltage  vq (pu)>"
  Bus Selector1/1 -> Gain/1, Steam Turbine and Governor/3  "<Rotor speed  wm  (pu)>"
  Bus Selector1/3 -> Excitation System/2  "<Stator voltage  vd (pu)>"
  Excitation System/1 -> Synchronous Machine pu Standard/2
  wref1/1 -> Excitation System/1
  Synchronous Machine pu Standard/1 -> Bus Selector1/1
  wref3/1 -> Steam Turbine and Governor/1
  wref2/1 -> Steam Turbine and Governor/2
  Bus Selector1/4 -> Steam Turbine and Governor/4  "<Rotor mechanical angle  theta (deg)>"
  Steam Turbine and Governor/3 -> Losses1/1, Synchronous Machine pu Standard/1
  Ground1/1 -> Excitation System/4
  connections:
  B/2/RConn1 -- Synchronous Machine pu Standard/RConn1 -- Load B2/LConn1 -- B/1/RConn1 -- Conn1/RConn1
  Synchronous Machine pu Standard/RConn2 -- B/1/RConn2 -- Conn2/RConn1 -- B/2/RConn2 -- Load B2/LConn2
  Synchronous Machine pu Standard/RConn3 -- B/1/RConn3 -- Conn3/RConn1 -- B/2/RConn3 -- Load B2/LConn3

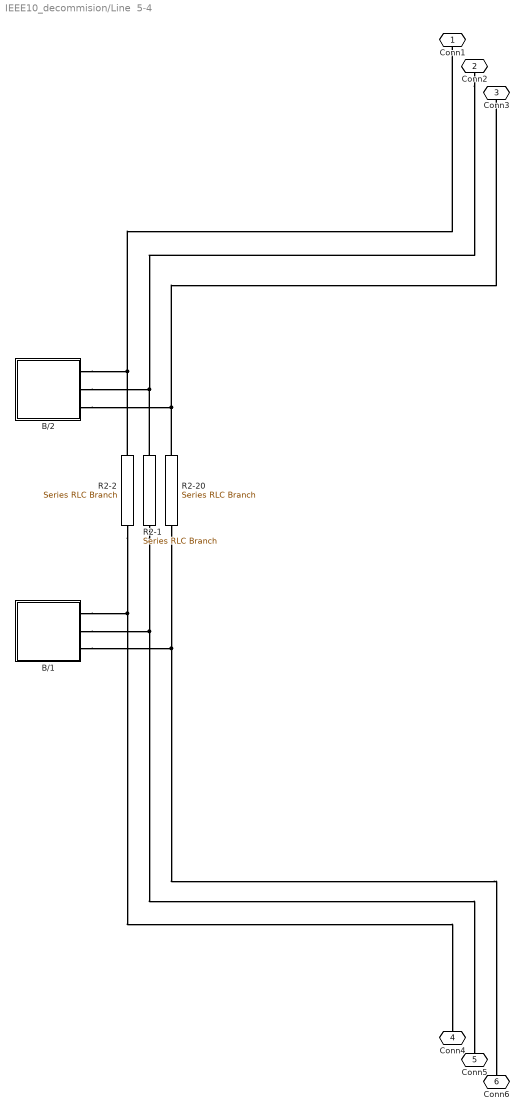
== system IEEE10_decommision/Line  5-4 ==
  B/1 : Subsystem
  B/2 : Subsystem
  R2-1 : powerlib/Elements/Series RLC Branch  LConnTagsString=__new0  RConnTagsString=__new0  BranchType=RL  Resistance=0.01*Xbase  Inductance=0.085*Lbase  SetiL0=off  InitialCurrent=0  Capacitance=1e-6  Setx0=off  InitialVoltage=0  Measurements=None
  R2-2 : powerlib/Elements/Series RLC Branch  LConnTagsString=__new0  RConnTagsString=__new0  BranchType=RL  Resistance=0.01*Xbase  Inductance=0.085*Lbase  SetiL0=off  InitialCurrent=0  Capacitance=1e-6  Setx0=off  InitialVoltage=0  Measurements=None
  R2-20 : powerlib/Elements/Series RLC Branch  LConnTagsString=__new0  RConnTagsString=__new0  BranchType=RL  Resistance=0.01*Xbase  Inductance=0.085*Lbase  SetiL0=off  InitialCurrent=0  Capacitance=1e-6  Setx0=off  InitialVoltage=0  Measurements=None
  Conn1 : PMIOPort  Port=1  Side=Right
  Conn2 : PMIOPort  Port=2  Side=Right
  Conn3 : PMIOPort  Port=3  Side=Right
  Conn4 : PMIOPort  Port=4  Side=Left
  Conn5 : PMIOPort  Port=5  Side=Left
  Conn6 : PMIOPort  Port=6  Side=Left
  connections:
  B/1/RConn1 -- Conn4/RConn1 -- R2-2/RConn1
  R2-20/RConn1 -- Conn6/RConn1 -- B/1/RConn3
  Conn2/RConn1 -- R2-1/LConn1 -- B/2/RConn2
  B/2/RConn1 -- R2-2/LConn1 -- Conn1/RConn1
  R2-20/LConn1 -- B/2/RConn3 -- Conn3/RConn1
  B/1/RConn2 -- Conn5/RConn1 -- R2-1/RConn1

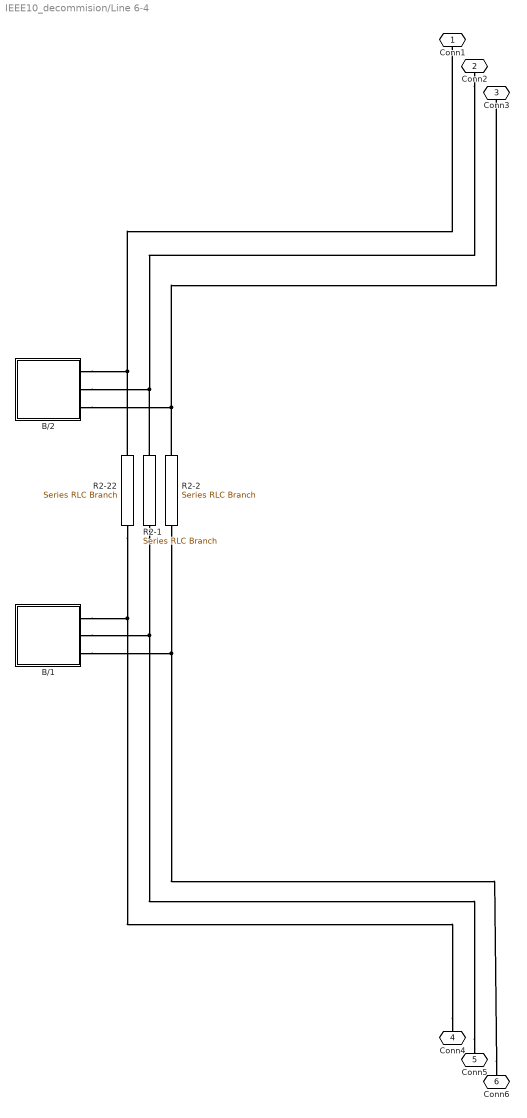
== system IEEE10_decommision/Line 6-4 ==
  B/1 : Subsystem
  B/2 : Subsystem
  R2-1 : powerlib/Elements/Series RLC Branch  LConnTagsString=__new0  RConnTagsString=__new0  BranchType=RL  Resistance=0.017*Xbase  Inductance=0.092*Lbase  SetiL0=off  InitialCurrent=0  Capacitance=1e-6  Setx0=off  InitialVoltage=0  Measurements=None
  R2-2 : powerlib/Elements/Series RLC Branch  LConnTagsString=__new0  RConnTagsString=__new0  BranchType=RL  Resistance=0.017*Xbase  Inductance=0.092*Lbase  SetiL0=off  InitialCurrent=0  Capacitance=1e-6  Setx0=off  InitialVoltage=0  Measurements=None
  R2-22 : powerlib/Elements/Series RLC Branch  LConnTagsString=__new0  RConnTagsString=__new0  BranchType=RL  Resistance=0.017*Xbase  Inductance=0.092*Lbase  SetiL0=off  InitialCurrent=0  Capacitance=1e-6  Setx0=off  InitialVoltage=0  Measurements=None
  Conn1 : PMIOPort  Port=1  Side=Right
  Conn2 : PMIOPort  Port=2  Side=Right
  Conn3 : PMIOPort  Port=3  Side=Right
  Conn4 : PMIOPort  Port=4  Side=Left
  Conn5 : PMIOPort  Port=5  Side=Left
  Conn6 : PMIOPort  Port=6  Side=Left
  connections:
  Conn5/RConn1 -- B/1/RConn2 -- R2-1/RConn1
  Conn3/RConn1 -- R2-2/LConn1 -- B/2/RConn3
  Conn1/RConn1 -- B/2/RConn1 -- R2-22/LConn1
  B/2/RConn2 -- R2-1/LConn1 -- Conn2/RConn1
  Conn6/RConn1 -- B/1/RConn3 -- R2-2/RConn1
  Conn4/RConn1 -- B/1/RConn1 -- R2-22/RConn1

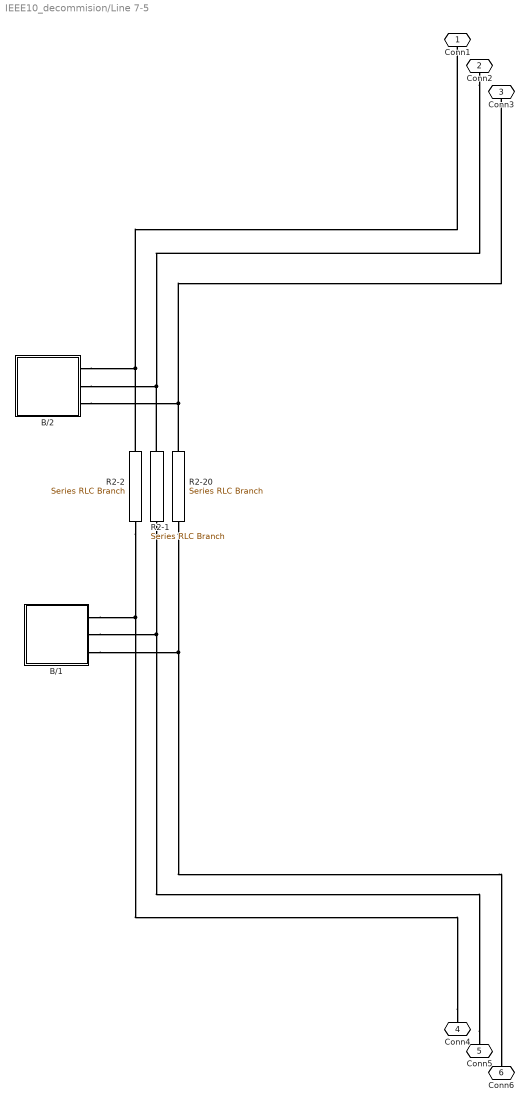
== system IEEE10_decommision/Line 7-5 ==
  B/1 : Subsystem
  B/2 : Subsystem
  R2-1 : powerlib/Elements/Series RLC Branch  LConnTagsString=__new0  RConnTagsString=__new0  BranchType=RL  Resistance=0.0032*Xbase  Inductance=0.161*Lbase  SetiL0=off  InitialCurrent=0  Capacitance=1e-6  Setx0=off  InitialVoltage=0  Measurements=None
  R2-2 : powerlib/Elements/Series RLC Branch  LConnTagsString=__new0  RConnTagsString=__new0  BranchType=RL  Resistance=0.0032*Xbase  Inductance=0.161*Lbase  SetiL0=off  InitialCurrent=0  Capacitance=1e-6  Setx0=off  InitialVoltage=0  Measurements=None
  R2-20 : powerlib/Elements/Series RLC Branch  LConnTagsString=__new0  RConnTagsString=__new0  BranchType=RL  Resistance=0.0032*Xbase  Inductance=0.161*Lbase  SetiL0=off  InitialCurrent=0  Capacitance=1e-6  Setx0=off  InitialVoltage=0  Measurements=None
  Conn1 : PMIOPort  Port=1  Side=Right
  Conn2 : PMIOPort  Port=2  Side=Right
  Conn3 : PMIOPort  Port=3  Side=Right
  Conn4 : PMIOPort  Port=4  Side=Left
  Conn5 : PMIOPort  Port=5  Side=Left
  Conn6 : PMIOPort  Port=6  Side=Left
  connections:
  Conn4/RConn1 -- B/1/RConn1 -- R2-2/RConn1
  R2-20/RConn1 -- B/1/RConn3 -- Conn6/RConn1
  Conn2/RConn1 -- B/2/RConn2 -- R2-1/LConn1
  R2-2/LConn1 -- B/2/RConn1 -- Conn1/RConn1
  R2-20/LConn1 -- B/2/RConn3 -- Conn3/RConn1
  Conn5/RConn1 -- B/1/RConn2 -- R2-1/RConn1

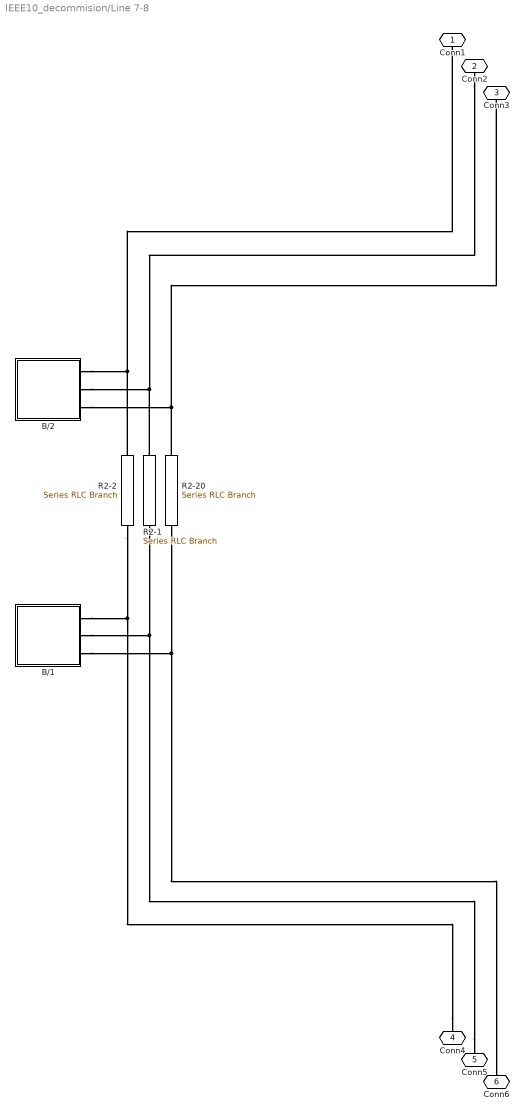
== system IEEE10_decommision/Line 7-8 ==
  B/1 : Subsystem
  B/2 : Subsystem
  R2-1 : powerlib/Elements/Series RLC Branch  LConnTagsString=__new0  RConnTagsString=__new0  BranchType=RL  Resistance=0.0085*Xbase  Inductance=0.072*Lbase  SetiL0=off  InitialCurrent=0  Capacitance=1e-6  Setx0=off  InitialVoltage=0  Measurements=None
  R2-2 : powerlib/Elements/Series RLC Branch  LConnTagsString=__new0  RConnTagsString=__new0  BranchType=RL  Resistance=0.0085*Xbase  Inductance=0.072*Lbase  SetiL0=off  InitialCurrent=0  Capacitance=1e-6  Setx0=off  InitialVoltage=0  Measurements=None
  R2-20 : powerlib/Elements/Series RLC Branch  LConnTagsString=__new0  RConnTagsString=__new0  BranchType=RL  Resistance=0.0085*Xbase  Inductance=0.072*Lbase  SetiL0=off  InitialCurrent=0  Capacitance=1e-6  Setx0=off  InitialVoltage=0  Measurements=None
  Conn1 : PMIOPort  Port=1  Side=Right
  Conn2 : PMIOPort  Port=2  Side=Right
  Conn3 : PMIOPort  Port=3  Side=Right
  Conn4 : PMIOPort  Port=4  Side=Left
  Conn5 : PMIOPort  Port=5  Side=Left
  Conn6 : PMIOPort  Port=6  Side=Left
  connections:
  Conn4/RConn1 -- B/1/RConn1 -- R2-2/RConn1
  R2-20/RConn1 -- B/1/RConn3 -- Conn6/RConn1
  Conn2/RConn1 -- R2-1/LConn1 -- B/2/RConn2
  B/2/RConn1 -- R2-2/LConn1 -- Conn1/RConn1
  R2-20/LConn1 -- B/2/RConn3 -- Conn3/RConn1
  Conn5/RConn1 -- B/1/RConn2 -- R2-1/RConn1

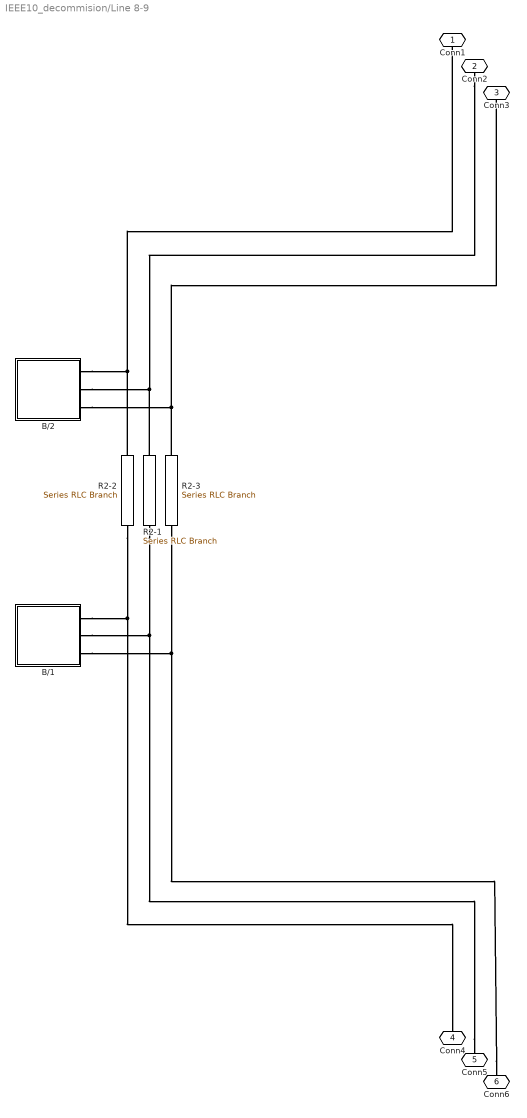
== system IEEE10_decommision/Line 8-9 ==
  B/1 : Subsystem
  B/2 : Subsystem
  R2-1 : powerlib/Elements/Series RLC Branch  LConnTagsString=__new0  RConnTagsString=__new0  BranchType=RL  Resistance=0.0119*Xbase  Inductance=0.1008*Lbase  SetiL0=off  InitialCurrent=0  Capacitance=1e-6  Setx0=off  InitialVoltage=0  Measurements=None
  R2-2 : powerlib/Elements/Series RLC Branch  LConnTagsString=__new0  RConnTagsString=__new0  BranchType=RL  Resistance=0.0119*Xbase  Inductance=0.1008*Lbase  SetiL0=off  InitialCurrent=0  Capacitance=1e-6  Setx0=off  InitialVoltage=0  Measurements=None
  R2-3 : powerlib/Elements/Series RLC Branch  LConnTagsString=__new0  RConnTagsString=__new0  BranchType=RL  Resistance=0.0119*Xbase  Inductance=0.1008*Lbase  SetiL0=off  InitialCurrent=0  Capacitance=1e-6  Setx0=off  InitialVoltage=0  Measurements=None
  Conn1 : PMIOPort  Port=1  Side=Right
  Conn2 : PMIOPort  Port=2  Side=Right
  Conn3 : PMIOPort  Port=3  Side=Right
  Conn4 : PMIOPort  Port=4  Side=Left
  Conn5 : PMIOPort  Port=5  Side=Left
  Conn6 : PMIOPort  Port=6  Side=Left
  connections:
  Conn5/RConn1 -- B/1/RConn2 -- R2-1/RConn1
  Conn3/RConn1 -- R2-3/LConn1 -- B/2/RConn3
  Conn1/RConn1 -- R2-2/LConn1 -- B/2/RConn1
  B/2/RConn2 -- R2-1/LConn1 -- Conn2/RConn1
  Conn6/RConn1 -- B/1/RConn3 -- R2-3/RConn1
  R2-2/RConn1 -- B/1/RConn1 -- Conn4/RConn1

== system IEEE10_decommision/Line 9-6 ==
  B/1 : Subsystem
  B/2 : Subsystem
  R2-1 : powerlib/Elements/Series RLC Branch  LConnTagsString=__new0  RConnTagsString=__new0  BranchType=RL  Resistance=0.039*Xbase  Inductance=0.17*Lbase  SetiL0=off  InitialCurrent=0  Capacitance=1e-6  Setx0=off  InitialVoltage=0  Measurements=None
  R2-2 : powerlib/Elements/Series RLC Branch  LConnTagsString=__new0  RConnTagsString=__new0  BranchType=RL  Resistance=0.039*Xbase  Inductance=0.17*Lbase  SetiL0=off  InitialCurrent=0  Capacitance=1e-6  Setx0=off  InitialVoltage=0  Measurements=None
  R2-20 : powerlib/Elements/Series RLC Branch  LConnTagsString=__new0  RConnTagsString=__new0  BranchType=RL  Resistance=0.039*Xbase  Inductance=0.17*Lbase  SetiL0=off  InitialCurrent=0  Capacitance=1e-6  Setx0=off  InitialVoltage=0  Measurements=None
  Conn1 : PMIOPort  Port=1  Side=Right
  Conn2 : PMIOPort  Port=2  Side=Right
  Conn3 : PMIOPort  Port=3  Side=Right
  Conn4 : PMIOPort  Port=4  Side=Left
  Conn5 : PMIOPort  Port=5  Side=Left
  Conn6 : PMIOPort  Port=6  Side=Left
  connections:
  B/1/RConn2 -- Conn5/RConn1 -- R2-1/RConn1
  Conn3/RConn1 -- B/2/RConn3 -- R2-20/LConn1
  Conn1/RConn1 -- R2-2/LConn1 -- B/2/RConn1
  B/2/RConn2 -- R2-1/LConn1 -- Conn2/RConn1
  B/1/RConn3 -- Conn6/RConn1 -- R2-20/RConn1
  B/1/RConn1 -- Conn4/RConn1 -- R2-2/RConn1

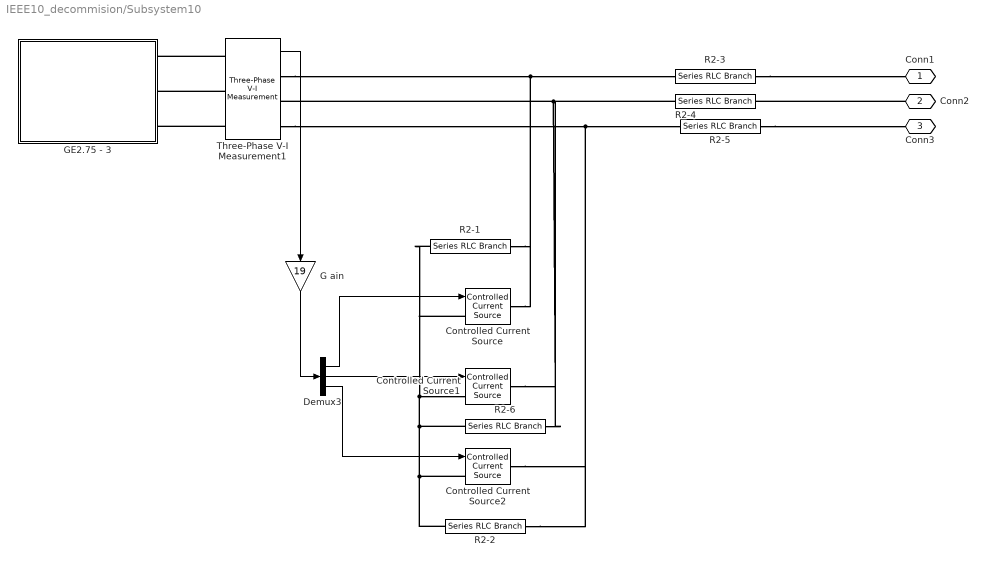
== system IEEE10_decommision/Subsystem10 ==
  Controlled Current Source : powerlib/Electrical Sources/Controlled Current Source  Initialize=off  Source_Type=AC  Amplitude=0  Phase=0  Frequency=0  Measurements=None
  Controlled Current Source1 : powerlib/Electrical Sources/Controlled Current Source  Initialize=off  Source_Type=AC  Amplitude=0  Phase=0  Frequency=0  Measurements=None
  Controlled Current Source2 : powerlib/Electrical Sources/Controlled Current Source  Initialize=off  Source_Type=AC  Amplitude=0  Phase=0  Frequency=0  Measurements=None
  Demux3 : Demux  Outputs=3
  G ain : Gain  Gain=19
  GE2.75 - 3 : Subsystem  mask{Prated=2.75e6, R=51.5, windspeed=9, Jtotal=1058.2, p=1.225, startuptime=5, winit=-166, gear=117.4, wmax=2*pi*(1735/60), fluxlinkage=4, pgen=2, Ld=10e-4, Lq=10.5e-4, Rs=1e-10, drivefreq=10e3, fnom=50, Srated=3.04e6, Vdcset=2500, Cdc=27e-3, Lfilter=2e-4, H=5, insup=50, supduration=5}
      mask prompts: Prated "Turbine Power (W)"; R "Blade Radius"; windspeed "Wind Speed"; Jtotal "Total Inertia"; p "Air Density"; startuptime "Turbine Start-up Time"; winit "Initial Generator Speed"; gear "Gearbox Ratio"; wmax "Max Generator Speed"; fluxlinkage "Flux Linkage"; pgen "Generator Pole Pairs"; Ld "Ld (H)"; Lq "Lq(H)"; Rs "Stator Resistance"; drivefreq "Drive Frequency"; fnom "Nominal Grid Frequency"; Srated "Drive Apparent Power"; Vdcset "DC Link Voltage"; Cdc "DC Link Capacitance"; Lfilter "Lfilter (H)"; H "Inertia Constant"; insup "Support Time"; supduration "Support Duration"
      mask Display: image(imread('gepic.jpg'))
  R2-1 : powerlib/Elements/Series RLC Branch  LConnTagsString=__new0  RConnTagsString=__new0  BranchType=R  Resistance=10000000  Inductance=1e-3  SetiL0=off  InitialCurrent=0  Capacitance=1000000*Cbase  Setx0=off  InitialVoltage=0  Measurements=None
  R2-2 : powerlib/Elements/Series RLC Branch  LConnTagsString=__new0  RConnTagsString=__new0  BranchType=R  Resistance=10000000  Inductance=1e-3  SetiL0=off  InitialCurrent=0  Capacitance=1000000*Cbase  Setx0=off  InitialVoltage=0  Measurements=None
  R2-3 : powerlib/Elements/Series RLC Branch  LConnTagsString=__new0  RConnTagsString=__new0  BranchType=R  Resistance=0.001  Inductance=1e-3  SetiL0=off  InitialCurrent=0  Capacitance=1000000*Cbase  Setx0=off  InitialVoltage=0  Measurements=None
  R2-4 : powerlib/Elements/Series RLC Branch  LConnTagsString=__new0  RConnTagsString=__new0  BranchType=R  Resistance=0.001  Inductance=1e-3  SetiL0=off  InitialCurrent=0  Capacitance=1000000*Cbase  Setx0=off  InitialVoltage=0  Measurements=None
  R2-5 : powerlib/Elements/Series RLC Branch  LConnTagsString=__new0  RConnTagsString=__new0  BranchType=R  Resistance=0.001  Inductance=1e-3  SetiL0=off  InitialCurrent=0  Capacitance=1000000*Cbase  Setx0=off  InitialVoltage=0  Measurements=None
  R2-6 : powerlib/Elements/Series RLC Branch  LConnTagsString=__new0  RConnTagsString=__new0  BranchType=R  Resistance=10000000  Inductance=1e-3  SetiL0=off  InitialCurrent=0  Capacitance=1000000*Cbase  Setx0=off  InitialVoltage=0  Measurements=None
  Three-Phase V-I Measurement1 : powerlib/Measurements/Three-Phase V-I Measurement  VoltageMeasurement=no  SetLabelV=off  LabelV=Vabc  Vpu=off  VpuLL=off  CurrentMeasurement=yes  SetLabelI=off  LabelI=Iabc  Ipu=off  Pbase=2.75e6  Vbase=690  OutputType=Complex  PhasorSimulation=off  PSBequivalent=0
  Conn1 : PMIOPort  Port=1  Side=Right
  Conn2 : PMIOPort  Port=2  Side=Right
  Conn3 : PMIOPort  Port=3  Side=Right
  wires:
  G ain/1 -> Demux3/1
  Three-Phase V-I Measurement1/1 -> G ain/1
  Demux3/1 -> Controlled Current Source/1
  Demux3/2 -> Controlled Current Source1/1
  Demux3/3 -> Controlled Current Source2/1
  connections:
  Controlled Current Source2/LConn1 -- R2-6/LConn1 -- R2-1/LConn1 -- Controlled Current Source/LConn1 -- Controlled Current Source1/LConn1 -- R2-2/LConn1
  Three-Phase V-I Measurement1/RConn1 -- R2-1/RConn1 -- Controlled Current Source/RConn1 -- R2-3/LConn1
  Three-Phase V-I Measurement1/LConn1 -- GE2.75 - 3/RConn1
  Three-Phase V-I Measurement1/LConn2 -- GE2.75 - 3/RConn2
  Three-Phase V-I Measurement1/LConn3 -- GE2.75 - 3/RConn3
  Three-Phase V-I Measurement1/RConn3 -- R2-2/RConn1 -- Controlled Current Source2/RConn1 -- R2-5/LConn1
  R2-3/RConn1 -- Conn1/RConn1
  Conn2/RConn1 -- R2-4/RConn1
  R2-5/RConn1 -- Conn3/RConn1
  R2-4/LConn1 -- R2-6/RConn1 -- Controlled Current Source1/RConn1 -- Three-Phase V-I Measurement1/RConn2

== system IEEE10_decommision/Gen 3/B//1 ==
  Ground : powerlib/Elements/Ground  LConnTagsString=a
  R2-1 : powerlib/Elements/Series RLC Branch  LConnTagsString=__new0  RConnTagsString=__new0  BranchType=R  Resistance=1000000  Inductance=1e-3  SetiL0=off  InitialCurrent=0  Capacitance=Cbase*0.088  Setx0=off  InitialVoltage=0  Measurements=None
  R2-2 : powerlib/Elements/Series RLC Branch  LConnTagsString=__new0  RConnTagsString=__new0  BranchType=R  Resistance=1000000  Inductance=1e-3  SetiL0=off  InitialCurrent=0  Capacitance=Cbase*0.088  Setx0=off  InitialVoltage=0  Measurements=None
  R2-3 : powerlib/Elements/Series RLC Branch  LConnTagsString=__new0  RConnTagsString=__new0  BranchType=R  Resistance=1000000  Inductance=1e-3  SetiL0=off  InitialCurrent=0  Capacitance=Cbase*0.088  Setx0=off  InitialVoltage=0  Measurements=None
  Conn1 : PMIOPort  Port=1  Side=Right
  Conn2 : PMIOPort  Port=2  Side=Right
  Conn3 : PMIOPort  Port=3  Side=Right
  connections:
  R2-2/LConn1 -- Conn1/RConn1
  R2-3/RConn1 -- R2-2/RConn1 -- R2-1/RConn1 -- Ground/LConn1
  R2-3/LConn1 -- Conn3/RConn1
  R2-1/LConn1 -- Conn2/RConn1

== system IEEE10_decommision/Gen 3/B//2 ==
  Ground : powerlib/Elements/Ground  LConnTagsString=a
  R2-1 : powerlib/Elements/Series RLC Branch  LConnTagsString=__new0  RConnTagsString=__new0  BranchType=R  Resistance=300  Inductance=1e-3  SetiL0=off  InitialCurrent=0  Capacitance=Cbase*0.088  Setx0=off  InitialVoltage=0  Measurements=None
  R2-2 : powerlib/Elements/Series RLC Branch  LConnTagsString=__new0  RConnTagsString=__new0  BranchType=R  Resistance=300  Inductance=1e-3  SetiL0=off  InitialCurrent=0  Capacitance=Cbase*0.088  Setx0=off  InitialVoltage=0  Measurements=None
  R2-3 : powerlib/Elements/Series RLC Branch  LConnTagsString=__new0  RConnTagsString=__new0  BranchType=R  Resistance=300  Inductance=1e-3  SetiL0=off  InitialCurrent=0  Capacitance=Cbase*0.088  Setx0=off  InitialVoltage=0  Measurements=None
  Conn1 : PMIOPort  Port=1  Side=Right
  Conn2 : PMIOPort  Port=2  Side=Right
  Conn3 : PMIOPort  Port=3  Side=Right
  connections:
  R2-1/LConn1 -- Conn2/RConn1
  R2-3/LConn1 -- Conn3/RConn1
  Ground/LConn1 -- R2-2/RConn1 -- R2-1/RConn1 -- R2-3/RConn1
  R2-2/LConn1 -- Conn1/RConn1

== system IEEE10_decommision/Gen1/B//1 ==
  Ground : powerlib/Elements/Ground  LConnTagsString=a
  R2-1 : powerlib/Elements/Series RLC Branch  LConnTagsString=__new0  RConnTagsString=__new0  BranchType=R  Resistance=1000000  Inductance=1e-3  SetiL0=off  InitialCurrent=0  Capacitance=Cbase*0.088  Setx0=off  InitialVoltage=0  Measurements=None
  R2-2 : powerlib/Elements/Series RLC Branch  LConnTagsString=__new0  RConnTagsString=__new0  BranchType=R  Resistance=1000000  Inductance=1e-3  SetiL0=off  InitialCurrent=0  Capacitance=Cbase*0.088  Setx0=off  InitialVoltage=0  Measurements=None
  R2-3 : powerlib/Elements/Series RLC Branch  LConnTagsString=__new0  RConnTagsString=__new0  BranchType=R  Resistance=1000000  Inductance=1e-3  SetiL0=off  InitialCurrent=0  Capacitance=Cbase*0.088  Setx0=off  InitialVoltage=0  Measurements=None
  Conn1 : PMIOPort  Port=1  Side=Right
  Conn2 : PMIOPort  Port=2  Side=Right
  Conn3 : PMIOPort  Port=3  Side=Right
  connections:
  R2-2/LConn1 -- Conn1/RConn1
  R2-2/RConn1 -- R2-3/RConn1 -- R2-1/RConn1 -- Ground/LConn1
  R2-3/LConn1 -- Conn3/RConn1
  R2-1/LConn1 -- Conn2/RConn1

== system IEEE10_decommision/Gen1/B//2 ==
  Ground : powerlib/Elements/Ground  LConnTagsString=a
  R2-1 : powerlib/Elements/Series RLC Branch  LConnTagsString=__new0  RConnTagsString=__new0  BranchType=R  Resistance=220  Inductance=1e-3  SetiL0=off  InitialCurrent=0  Capacitance=Cbase*0.088  Setx0=off  InitialVoltage=0  Measurements=None
  R2-2 : powerlib/Elements/Series RLC Branch  LConnTagsString=__new0  RConnTagsString=__new0  BranchType=R  Resistance=220  Inductance=1e-3  SetiL0=off  InitialCurrent=0  Capacitance=Cbase*0.088  Setx0=off  InitialVoltage=0  Measurements=None
  R2-3 : powerlib/Elements/Series RLC Branch  LConnTagsString=__new0  RConnTagsString=__new0  BranchType=R  Resistance=220  Inductance=1e-3  SetiL0=off  InitialCurrent=0  Capacitance=Cbase*0.088  Setx0=off  InitialVoltage=0  Measurements=None
  Conn1 : PMIOPort  Port=1  Side=Right
  Conn2 : PMIOPort  Port=2  Side=Right
  Conn3 : PMIOPort  Port=3  Side=Right
  connections:
  R2-1/LConn1 -- Conn2/RConn1
  R2-3/LConn1 -- Conn3/RConn1
  Ground/LConn1 -- R2-2/RConn1 -- R2-1/RConn1 -- R2-3/RConn1
  R2-2/LConn1 -- Conn1/RConn1

== system IEEE10_decommision/Gen2/B//1 ==
  Ground : powerlib/Elements/Ground  LConnTagsString=a
  R2-1 : powerlib/Elements/Series RLC Branch  LConnTagsString=__new0  RConnTagsString=__new0  BranchType=R  Resistance=1000000  Inductance=1e-3  SetiL0=off  InitialCurrent=0  Capacitance=Cbase*0.088  Setx0=off  InitialVoltage=0  Measurements=None
  R2-2 : powerlib/Elements/Series RLC Branch  LConnTagsString=__new0  RConnTagsString=__new0  BranchType=R  Resistance=1000000  Inductance=1e-3  SetiL0=off  InitialCurrent=0  Capacitance=Cbase*0.088  Setx0=off  InitialVoltage=0  Measurements=None
  R2-3 : powerlib/Elements/Series RLC Branch  LConnTagsString=__new0  RConnTagsString=__new0  BranchType=R  Resistance=1000000  Inductance=1e-3  SetiL0=off  InitialCurrent=0  Capacitance=Cbase*0.088  Setx0=off  InitialVoltage=0  Measurements=None
  Conn1 : PMIOPort  Port=1  Side=Right
  Conn2 : PMIOPort  Port=2  Side=Right
  Conn3 : PMIOPort  Port=3  Side=Right
  connections:
  R2-2/LConn1 -- Conn1/RConn1
  R2-2/RConn1 -- R2-3/RConn1 -- R2-1/RConn1 -- Ground/LConn1
  R2-3/LConn1 -- Conn3/RConn1
  R2-1/LConn1 -- Conn2/RConn1

== system IEEE10_decommision/Gen2/B//2 ==
  Ground : powerlib/Elements/Ground  LConnTagsString=a
  R2-1 : powerlib/Elements/Series RLC Branch  LConnTagsString=__new0  RConnTagsString=__new0  BranchType=R  Resistance=324  Inductance=1e-3  SetiL0=off  InitialCurrent=0  Capacitance=Cbase*0.088  Setx0=off  InitialVoltage=0  Measurements=None
  R2-2 : powerlib/Elements/Series RLC Branch  LConnTagsString=__new0  RConnTagsString=__new0  BranchType=R  Resistance=324  Inductance=1e-3  SetiL0=off  InitialCurrent=0  Capacitance=Cbase*0.088  Setx0=off  InitialVoltage=0  Measurements=None
  R2-3 : powerlib/Elements/Series RLC Branch  LConnTagsString=__new0  RConnTagsString=__new0  BranchType=R  Resistance=324  Inductance=1e-3  SetiL0=off  InitialCurrent=0  Capacitance=Cbase*0.088  Setx0=off  InitialVoltage=0  Measurements=None
  Conn1 : PMIOPort  Port=1  Side=Right
  Conn2 : PMIOPort  Port=2  Side=Right
  Conn3 : PMIOPort  Port=3  Side=Right
  connections:
  R2-1/LConn1 -- Conn2/RConn1
  R2-3/LConn1 -- Conn3/RConn1
  Ground/LConn1 -- R2-2/RConn1 -- R2-1/RConn1 -- R2-3/RConn1
  R2-2/LConn1 -- Conn1/RConn1
